simulink model "mining_feeder_layer_FDIR"  (R2024a)
settings: Solver=ode23t  StartTime=0.0  StopTime=2.0  FixedStep=5e-06  MaxStep=0.001  RelTol=1e-3
undefined symbols (not defined in the file or in its folder): D11, Delta, gcbh, Newton, Raphson, sps_rtmsupport
libraries: spsFourierLib x8, spsMeanLib x8, spsThreePhaseVIMeasurementLib x7, spsRMSLib x6, spsThreePhaseBreakerLib x5, spsThreePhaseSeriesRLCLoadLib x4, spsThreePhaseFaultLib x4, spsThreePhasePISectionLineLib x4, spsThreePhaseTransformerTwoWindingsLib x2, spsThreePhaseSourceLib x1, sps_lib x1
settings Model: Creator=victo  LastModifiedBy=victo

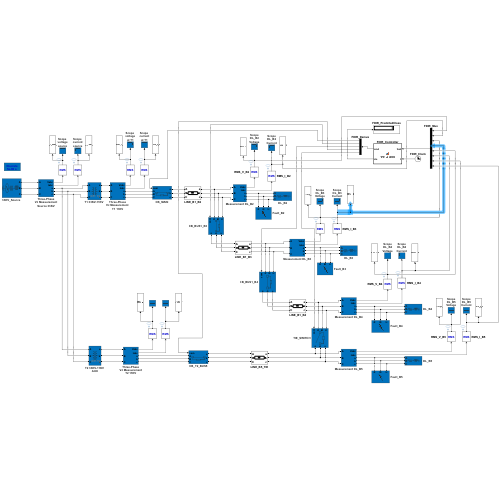
[thumbnail: Simulink's stored preview of the top-level diagram]
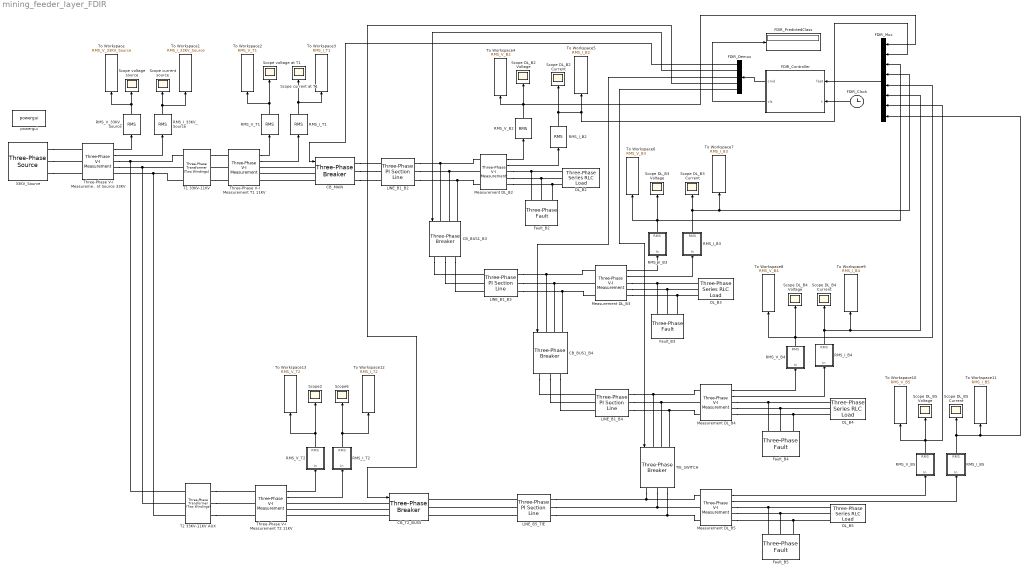
== system mining_feeder_layer_FDIR ==
  "33KV_Source " : spsThreePhaseSourceLib/Three-Phase Source  InternalConnection=Yg  VoltagePhases=off  Voltage=33e3  PhaseAngle=0  Voltage_phases=[25e3 25e3 25e3]/sqrt(3)  PhaseAngles_phases=[0 -120 +120]  Frequency=50  NonIdealSource=on  SpecifyImpedance=on  Resistance=0.8929  Inductance=16.58e-3  ShortCircuitLevel=500e6  BaseVoltage=33e3  XRratio=10  BusType=swing  Pref=10e3  Qref=0  Prefabc=[10e3, 10e3, 10e3]  Qrefabc=[0, 0, 0]  Qmin=-inf  Qmax=inf
  CB_BUS1_B3 : spsThreePhaseBreakerLib/Three-Phase Breaker  InitialState=closed  SwitchA=on  SwitchB=on  SwitchC=on  SwitchTimes=[1000000 1000001]  External=on  BreakerResistance=0.01  SnubberResistance=1e5  SnubberCapacitance=1e-9  Measurements=None
  CB_BUS1_B4 : spsThreePhaseBreakerLib/Three-Phase Breaker  InitialState=closed  SwitchA=on  SwitchB=on  SwitchC=on  SwitchTimes=[1000000 1000001]  External=on  BreakerResistance=0.01  SnubberResistance=1e5  SnubberCapacitance=1e-9  Measurements=None
  CB_MAIN : spsThreePhaseBreakerLib/Three-Phase Breaker  InitialState=closed  SwitchA=on  SwitchB=on  SwitchC=on  SwitchTimes=[1000000 1000001]  External=on  BreakerResistance=0.01  SnubberResistance=1e6  SnubberCapacitance=inf  Measurements=None
  CB_T2_BUS5 : spsThreePhaseBreakerLib/Three-Phase Breaker  InitialState=closed  SwitchA=on  SwitchB=on  SwitchC=on  SwitchTimes=[1000000 1000001]  External=on  BreakerResistance=0.01  SnubberResistance=1e5  SnubberCapacitance=1e-9  Measurements=None
  DL_B2 : spsThreePhaseSeriesRLCLoadLib/Three-Phase Series RLC Load  LConnTagsString=A|B|C  Configuration=Y (grounded)  NominalVoltage=11e3  Vabc=[1e3 1e3 1e3]  Vabcp=[1e3 1e3 1e3]  NominalFrequency=50  UnbalancedPower=off  ActivePower=2340000  InductivePower=572000  CapacitivePower=0  Pabc=[10e3 9e3 11e3]  QLabc=[100 90 110]  QCabc=[100 90 110]  Pabcp=[10e3 9e3 11e3]  QLabcp=[100 90 110]  QCabcp=[100 90 110]  Measurements=None  LoadType=constant Z
  DL_B3 : spsThreePhaseSeriesRLCLoadLib/Three-Phase Series RLC Load  LConnTagsString=A|B|C  Configuration=Y (grounded)  NominalVoltage=11e3  Vabc=[1e3 1e3 1e3]  Vabcp=[1e3 1e3 1e3]  NominalFrequency=50  UnbalancedPower=off  ActivePower=3120000  InductivePower=767000  CapacitivePower=0  Pabc=[10e3 9e3 11e3]  QLabc=[100 90 110]  QCabc=[100 90 110]  Pabcp=[10e3 9e3 11e3]  QLabcp=[100 90 110]  QCabcp=[100 90 110]  Measurements=None  LoadType=constant Z
  DL_B4 : spsThreePhaseSeriesRLCLoadLib/Three-Phase Series RLC Load  LConnTagsString=A|B|C  Configuration=Y (grounded)  NominalVoltage=11e3  Vabc=[1e3 1e3 1e3]  Vabcp=[1e3 1e3 1e3]  NominalFrequency=50  UnbalancedPower=off  ActivePower=3900000  InductivePower=962000  CapacitivePower=0  Pabc=[10e3 9e3 11e3]  QLabc=[100 90 110]  QCabc=[100 90 110]  Pabcp=[10e3 9e3 11e3]  QLabcp=[100 90 110]  QCabcp=[100 90 110]  Measurements=None  LoadType=constant Z
  DL_B5 : spsThreePhaseSeriesRLCLoadLib/Three-Phase Series RLC Load  LConnTagsString=A|B|C  Configuration=Y (grounded)  NominalVoltage=11e3  Vabc=[1e3 1e3 1e3]  Vabcp=[1e3 1e3 1e3]  NominalFrequency=50  UnbalancedPower=off  ActivePower=2574000  InductivePower=637000  CapacitivePower=0  Pabc=[10e3 9e3 11e3]  QLabc=[100 90 110]  QCabc=[100 90 110]  Pabcp=[10e3 9e3 11e3]  QLabcp=[100 90 110]  QCabcp=[100 90 110]  Measurements=None  LoadType=constant Z
  FDIR_Clock : Clock
  FDIR_Controller : MATLAB Function  TreatAsAtomicUnit=on
  FDIR_Demux : Demux  Outputs=5
  FDIR_Mux : Mux  Inputs=8
  FDIR_PredictedClass : Display
  Fault_B2 : spsThreePhaseFaultLib/Three-Phase Fault  InitialStates=0  FaultA=off  FaultB=off  FaultC=off  GroundFault=off  SwitchTimes=[100000 100001]  External=off  SwitchStatus=NaN  FaultResistance=0.001  GroundResistance=0.001  SnubberResistance=1e5  SnubberCapacitance=1e-9  Measurements=None
  Fault_B3 : spsThreePhaseFaultLib/Three-Phase Fault  InitialStates=0  FaultA=off  FaultB=off  FaultC=off  GroundFault=off  SwitchTimes=[1000000 1000001]  External=off  SwitchStatus=NaN  FaultResistance=0.001  GroundResistance=0.001  SnubberResistance=1e5  SnubberCapacitance=1e-9  Measurements=None
  Fault_B4 : spsThreePhaseFaultLib/Three-Phase Fault  InitialStates=0  FaultA=off  FaultB=off  FaultC=off  GroundFault=off  SwitchTimes=[1000000 1000001]  External=off  SwitchStatus=NaN  FaultResistance=0.001  GroundResistance=0.001  SnubberResistance=1e5  SnubberCapacitance=1e-9  Measurements=None
  Fault_B5 : spsThreePhaseFaultLib/Three-Phase Fault  InitialStates=0  FaultA=off  FaultB=off  FaultC=off  GroundFault=off  SwitchTimes=[1000000 1000001]  External=off  SwitchStatus=NaN  FaultResistance=0.001  GroundResistance=0.001  SnubberResistance=1e5  SnubberCapacitance=1e-9  Measurements=None
  LINE_B1_B2 : spsThreePhasePISectionLineLib/Three-Phase PI Section Line  LConnTagsString=a|b|c  RConnTagsString=A|B|C  Length=0.8  Frequency=50  Resistances=[0.12 0.36]  Inductances=[0.35e-3 1.05e-3]  Capacitances=[0.20e-6 0.10e-6]
  LINE_B1_B3 : spsThreePhasePISectionLineLib/Three-Phase PI Section Line  LConnTagsString=a|b|c  RConnTagsString=A|B|C  Length=1.2  Frequency=50  Resistances=[0.12 0.36]  Inductances=[0.35e-3 1.05e-3]  Capacitances=[0.20e-6 0.10e-6]
  LINE_B1_B4 : spsThreePhasePISectionLineLib/Three-Phase PI Section Line  LConnTagsString=a|b|c  RConnTagsString=A|B|C  Length=1.0  Frequency=50  Resistances=[0.12 0.36]  Inductances=[0.35e-3 1.05e-3]  Capacitances=[0.20e-6 0.10e-6]
  LINE_B5_TIE : spsThreePhasePISectionLineLib/Three-Phase PI Section Line  LConnTagsString=a|b|c  RConnTagsString=A|B|C  Length=0.6  Frequency=50  Resistances=[0.12 0.36]  Inductances=[0.35e-3 1.05e-3]  Capacitances=[0.20e-6 0.10e-6]
  Measurement DL_B{2..5} (4 alike) : spsThreePhaseVIMeasurementLib/Three-Phase V-I Measurement  VoltageMeasurement=phase-to-phase  SetLabelV=off  LabelV=Vabc  Vpu=off  VpuLL=off  CurrentMeasurement=yes  SetLabelI=off  LabelI=Iabc  Ipu=off  Pbase=100e6  Vbase=500e3  OutputType=Complex  PhasorSimulation=off  PSBequivalent=0
  RMS_I_33KV_Source : spsRMSLib/RMS  TrueRMS=on  Freq=50  RMSInit=0  Ts=0.0001
  RMS_I_B2 : spsRMSLib/RMS  TrueRMS=on  Freq=50  RMSInit=50  Ts=0.0001
  RMS_I_B3 : Subsystem  DialogController=POWERSYS.PowerSysDialog  LoadFcn=sps_rtmsupport('LoadFcn', gcbh);  StartFcn=sps_rtmsupport('StartFcn', gcbh);  StopFcn=sps_rtmsupport('StopFcn', gcbh);  mask(RMS){TrueRMS=on, Freq=50, RMSInit=0, Ts=0.0001}
      mask prompts: TrueRMS "True RMS value"; Freq "Fundamental frequency (Hz):"; RMSInit "Initial RMS value:"; Ts "Sample time:"
      mask help:
      | Measure the true root mean square (RMS) value of the input signal at the specified fundamental frequency.
      |
      | When True RMS value parameter is unchecked, the block outputs the RMS value of the fundamental component of the input signal.
      mask init:
      | [sps] = powericon('RMSInit',gcb,Freq,RMSInit,TrueRMS,Ts);
      settings: LibrarySourceBlock=sps_lib/Sensors and Measurements/RMS  CopyFcn=sps_rtmsupport('CopyFcn', gcbh);  DeleteFcn=sps_rtmsupport('DeleteFcn', gcbh);  UndoDeleteFcn=sps_rtmsupport('UndoDeleteFcn', gcbh);  ModelCloseFcn=sps_rtmsupport('ModelCloseFcn', gcbh);  PreSaveFcn=sps_rtmsupport('PreSaveFcn', gcbh);  PostSaveFcn=sps_rtmsupport('PostSaveFcn', gcbh);  NameChangeFcn=sps_rtmsupport('NameChangeFcn', gcbh);  PreCopyFcn=sps_rtmsupport('PreCopyFcn', gcbh);  OpenFcn=sps_rtmsupport('OpenFcn', gcbh, [1]);  CloseFcn=sps_rtmsupport('CloseFcn', gcbh);  PreDeleteFcn=sps_rtmsupport('PreDeleteFcn', gcbh);
      mask Help: helpview(psbhelp);
      mask Display: color('blue');disp('RMS')
  RMS_I_B4 : Subsystem  DialogController=POWERSYS.PowerSysDialog  LoadFcn=sps_rtmsupport('LoadFcn', gcbh);  StartFcn=sps_rtmsupport('StartFcn', gcbh);  StopFcn=sps_rtmsupport('StopFcn', gcbh);  mask(RMS){TrueRMS=on, Freq=50, RMSInit=0, Ts=0.0001}
      mask prompts: TrueRMS "True RMS value"; Freq "Fundamental frequency (Hz):"; RMSInit "Initial RMS value:"; Ts "Sample time:"
      mask help:
      | Measure the true root mean square (RMS) value of the input signal at the specified fundamental frequency.
      |
      | When True RMS value parameter is unchecked, the block outputs the RMS value of the fundamental component of the input signal.
      mask init:
      | [sps] = powericon('RMSInit',gcb,Freq,RMSInit,TrueRMS,Ts);
      settings: LibrarySourceBlock=sps_lib/Sensors and Measurements/RMS  CopyFcn=sps_rtmsupport('CopyFcn', gcbh);  DeleteFcn=sps_rtmsupport('DeleteFcn', gcbh);  UndoDeleteFcn=sps_rtmsupport('UndoDeleteFcn', gcbh);  ModelCloseFcn=sps_rtmsupport('ModelCloseFcn', gcbh);  PreSaveFcn=sps_rtmsupport('PreSaveFcn', gcbh);  PostSaveFcn=sps_rtmsupport('PostSaveFcn', gcbh);  NameChangeFcn=sps_rtmsupport('NameChangeFcn', gcbh);  PreCopyFcn=sps_rtmsupport('PreCopyFcn', gcbh);  OpenFcn=sps_rtmsupport('OpenFcn', gcbh, [1]);  CloseFcn=sps_rtmsupport('CloseFcn', gcbh);  PreDeleteFcn=sps_rtmsupport('PreDeleteFcn', gcbh);
      mask Help: helpview(psbhelp);
      mask Display: color('blue');disp('RMS')
  RMS_I_B5 : Subsystem  DialogController=POWERSYS.PowerSysDialog  LoadFcn=sps_rtmsupport('LoadFcn', gcbh);  StartFcn=sps_rtmsupport('StartFcn', gcbh);  StopFcn=sps_rtmsupport('StopFcn', gcbh);  mask(RMS){TrueRMS=on, Freq=50, RMSInit=0, Ts=0.0001}
      mask prompts: TrueRMS "True RMS value"; Freq "Fundamental frequency (Hz):"; RMSInit "Initial RMS value:"; Ts "Sample time:"
      mask help:
      | Measure the true root mean square (RMS) value of the input signal at the specified fundamental frequency.
      |
      | When True RMS value parameter is unchecked, the block outputs the RMS value of the fundamental component of the input signal.
      mask init:
      | [sps] = powericon('RMSInit',gcb,Freq,RMSInit,TrueRMS,Ts);
      settings: LibrarySourceBlock=sps_lib/Sensors and Measurements/RMS  CopyFcn=sps_rtmsupport('CopyFcn', gcbh);  DeleteFcn=sps_rtmsupport('DeleteFcn', gcbh);  UndoDeleteFcn=sps_rtmsupport('UndoDeleteFcn', gcbh);  ModelCloseFcn=sps_rtmsupport('ModelCloseFcn', gcbh);  PreSaveFcn=sps_rtmsupport('PreSaveFcn', gcbh);  PostSaveFcn=sps_rtmsupport('PostSaveFcn', gcbh);  NameChangeFcn=sps_rtmsupport('NameChangeFcn', gcbh);  PreCopyFcn=sps_rtmsupport('PreCopyFcn', gcbh);  OpenFcn=sps_rtmsupport('OpenFcn', gcbh, [1]);  CloseFcn=sps_rtmsupport('CloseFcn', gcbh);  PreDeleteFcn=sps_rtmsupport('PreDeleteFcn', gcbh);
      mask Help: helpview(psbhelp);
      mask Display: color('blue');disp('RMS')
  RMS_I_T1 : spsRMSLib/RMS  TrueRMS=on  Freq=50  RMSInit=0  Ts=0.0001
  RMS_I_T2 : Subsystem  DialogController=POWERSYS.PowerSysDialog  LoadFcn=sps_rtmsupport('LoadFcn', gcbh);  StartFcn=sps_rtmsupport('StartFcn', gcbh);  StopFcn=sps_rtmsupport('StopFcn', gcbh);  mask(RMS){TrueRMS=on, Freq=50, RMSInit=0, Ts=0.0001}
      mask prompts: TrueRMS "True RMS value"; Freq "Fundamental frequency (Hz):"; RMSInit "Initial RMS value:"; Ts "Sample time:"
      mask help:
      | Measure the true root mean square (RMS) value of the input signal at the specified fundamental frequency.
      |
      | When True RMS value parameter is unchecked, the block outputs the RMS value of the fundamental component of the input signal.
      mask init:
      | [sps] = powericon('RMSInit',gcb,Freq,RMSInit,TrueRMS,Ts);
      settings: LibrarySourceBlock=sps_lib/Sensors and Measurements/RMS  CopyFcn=sps_rtmsupport('CopyFcn', gcbh);  DeleteFcn=sps_rtmsupport('DeleteFcn', gcbh);  UndoDeleteFcn=sps_rtmsupport('UndoDeleteFcn', gcbh);  ModelCloseFcn=sps_rtmsupport('ModelCloseFcn', gcbh);  PreSaveFcn=sps_rtmsupport('PreSaveFcn', gcbh);  PostSaveFcn=sps_rtmsupport('PostSaveFcn', gcbh);  NameChangeFcn=sps_rtmsupport('NameChangeFcn', gcbh);  PreCopyFcn=sps_rtmsupport('PreCopyFcn', gcbh);  OpenFcn=sps_rtmsupport('OpenFcn', gcbh, [1]);  CloseFcn=sps_rtmsupport('CloseFcn', gcbh);  PreDeleteFcn=sps_rtmsupport('PreDeleteFcn', gcbh);
      mask Help: helpview(psbhelp);
      mask Display: color('blue');disp('RMS')
  RMS_V_33KV_Source : spsRMSLib/RMS  TrueRMS=on  Freq=50  RMSInit=0  Ts=0.0001
  RMS_V_B2 : spsRMSLib/RMS  TrueRMS=on  Freq=50  RMSInit=9000  Ts=0.0001
  RMS_V_B3 : Subsystem  DialogController=POWERSYS.PowerSysDialog  LoadFcn=sps_rtmsupport('LoadFcn', gcbh);  StartFcn=sps_rtmsupport('StartFcn', gcbh);  StopFcn=sps_rtmsupport('StopFcn', gcbh);  mask(RMS){TrueRMS=on, Freq=50, RMSInit=0, Ts=0.0001}
      mask prompts: TrueRMS "True RMS value"; Freq "Fundamental frequency (Hz):"; RMSInit "Initial RMS value:"; Ts "Sample time:"
      mask help:
      | Measure the true root mean square (RMS) value of the input signal at the specified fundamental frequency.
      |
      | When True RMS value parameter is unchecked, the block outputs the RMS value of the fundamental component of the input signal.
      mask init:
      | [sps] = powericon('RMSInit',gcb,Freq,RMSInit,TrueRMS,Ts);
      settings: LibrarySourceBlock=sps_lib/Sensors and Measurements/RMS  CopyFcn=sps_rtmsupport('CopyFcn', gcbh);  DeleteFcn=sps_rtmsupport('DeleteFcn', gcbh);  UndoDeleteFcn=sps_rtmsupport('UndoDeleteFcn', gcbh);  ModelCloseFcn=sps_rtmsupport('ModelCloseFcn', gcbh);  PreSaveFcn=sps_rtmsupport('PreSaveFcn', gcbh);  PostSaveFcn=sps_rtmsupport('PostSaveFcn', gcbh);  NameChangeFcn=sps_rtmsupport('NameChangeFcn', gcbh);  PreCopyFcn=sps_rtmsupport('PreCopyFcn', gcbh);  OpenFcn=sps_rtmsupport('OpenFcn', gcbh, [1]);  CloseFcn=sps_rtmsupport('CloseFcn', gcbh);  PreDeleteFcn=sps_rtmsupport('PreDeleteFcn', gcbh);
      mask Help: helpview(psbhelp);
      mask Display: color('blue');disp('RMS')
  RMS_V_B4 : Subsystem  DialogController=POWERSYS.PowerSysDialog  LoadFcn=sps_rtmsupport('LoadFcn', gcbh);  StartFcn=sps_rtmsupport('StartFcn', gcbh);  StopFcn=sps_rtmsupport('StopFcn', gcbh);  mask(RMS){TrueRMS=on, Freq=50, RMSInit=0, Ts=0.0001}
      mask prompts: TrueRMS "True RMS value"; Freq "Fundamental frequency (Hz):"; RMSInit "Initial RMS value:"; Ts "Sample time:"
      mask help:
      | Measure the true root mean square (RMS) value of the input signal at the specified fundamental frequency.
      |
      | When True RMS value parameter is unchecked, the block outputs the RMS value of the fundamental component of the input signal.
      mask init:
      | [sps] = powericon('RMSInit',gcb,Freq,RMSInit,TrueRMS,Ts);
      settings: LibrarySourceBlock=sps_lib/Sensors and Measurements/RMS  CopyFcn=sps_rtmsupport('CopyFcn', gcbh);  DeleteFcn=sps_rtmsupport('DeleteFcn', gcbh);  UndoDeleteFcn=sps_rtmsupport('UndoDeleteFcn', gcbh);  ModelCloseFcn=sps_rtmsupport('ModelCloseFcn', gcbh);  PreSaveFcn=sps_rtmsupport('PreSaveFcn', gcbh);  PostSaveFcn=sps_rtmsupport('PostSaveFcn', gcbh);  NameChangeFcn=sps_rtmsupport('NameChangeFcn', gcbh);  PreCopyFcn=sps_rtmsupport('PreCopyFcn', gcbh);  OpenFcn=sps_rtmsupport('OpenFcn', gcbh, [1]);  CloseFcn=sps_rtmsupport('CloseFcn', gcbh);  PreDeleteFcn=sps_rtmsupport('PreDeleteFcn', gcbh);
      mask Help: helpview(psbhelp);
      mask Display: color('blue');disp('RMS')
  RMS_V_B5 : Subsystem  DialogController=POWERSYS.PowerSysDialog  LoadFcn=sps_rtmsupport('LoadFcn', gcbh);  StartFcn=sps_rtmsupport('StartFcn', gcbh);  StopFcn=sps_rtmsupport('StopFcn', gcbh);  mask(RMS){TrueRMS=on, Freq=50, RMSInit=0, Ts=0.0001}
      mask prompts: TrueRMS "True RMS value"; Freq "Fundamental frequency (Hz):"; RMSInit "Initial RMS value:"; Ts "Sample time:"
      mask help:
      | Measure the true root mean square (RMS) value of the input signal at the specified fundamental frequency.
      |
      | When True RMS value parameter is unchecked, the block outputs the RMS value of the fundamental component of the input signal.
      mask init:
      | [sps] = powericon('RMSInit',gcb,Freq,RMSInit,TrueRMS,Ts);
      settings: LibrarySourceBlock=sps_lib/Sensors and Measurements/RMS  CopyFcn=sps_rtmsupport('CopyFcn', gcbh);  DeleteFcn=sps_rtmsupport('DeleteFcn', gcbh);  UndoDeleteFcn=sps_rtmsupport('UndoDeleteFcn', gcbh);  ModelCloseFcn=sps_rtmsupport('ModelCloseFcn', gcbh);  PreSaveFcn=sps_rtmsupport('PreSaveFcn', gcbh);  PostSaveFcn=sps_rtmsupport('PostSaveFcn', gcbh);  NameChangeFcn=sps_rtmsupport('NameChangeFcn', gcbh);  PreCopyFcn=sps_rtmsupport('PreCopyFcn', gcbh);  OpenFcn=sps_rtmsupport('OpenFcn', gcbh, [1]);  CloseFcn=sps_rtmsupport('CloseFcn', gcbh);  PreDeleteFcn=sps_rtmsupport('PreDeleteFcn', gcbh);
      mask Help: helpview(psbhelp);
      mask Display: color('blue');disp('RMS')
  RMS_V_T1 : spsRMSLib/RMS  TrueRMS=on  Freq=50  RMSInit=0  Ts=0.0001
  RMS_V_T2 : Subsystem  DialogController=POWERSYS.PowerSysDialog  LoadFcn=sps_rtmsupport('LoadFcn', gcbh);  StartFcn=sps_rtmsupport('StartFcn', gcbh);  StopFcn=sps_rtmsupport('StopFcn', gcbh);  mask(RMS){TrueRMS=on, Freq=50, RMSInit=0, Ts=0.0001}
      mask prompts: TrueRMS "True RMS value"; Freq "Fundamental frequency (Hz):"; RMSInit "Initial RMS value:"; Ts "Sample time:"
      mask help:
      | Measure the true root mean square (RMS) value of the input signal at the specified fundamental frequency.
      |
      | When True RMS value parameter is unchecked, the block outputs the RMS value of the fundamental component of the input signal.
      mask init:
      | [sps] = powericon('RMSInit',gcb,Freq,RMSInit,TrueRMS,Ts);
      settings: LibrarySourceBlock=sps_lib/Sensors and Measurements/RMS  CopyFcn=sps_rtmsupport('CopyFcn', gcbh);  DeleteFcn=sps_rtmsupport('DeleteFcn', gcbh);  UndoDeleteFcn=sps_rtmsupport('UndoDeleteFcn', gcbh);  ModelCloseFcn=sps_rtmsupport('ModelCloseFcn', gcbh);  PreSaveFcn=sps_rtmsupport('PreSaveFcn', gcbh);  PostSaveFcn=sps_rtmsupport('PostSaveFcn', gcbh);  NameChangeFcn=sps_rtmsupport('NameChangeFcn', gcbh);  PreCopyFcn=sps_rtmsupport('PreCopyFcn', gcbh);  OpenFcn=sps_rtmsupport('OpenFcn', gcbh, [1]);  CloseFcn=sps_rtmsupport('CloseFcn', gcbh);  PreDeleteFcn=sps_rtmsupport('PreDeleteFcn', gcbh);
      mask Help: helpview(psbhelp);
      mask Display: color('blue');disp('RMS')
  Scope DL_B2 Current : Scope
  Scope DL_B2 Voltage : Scope
  Scope DL_B3 Current : Scope
  Scope DL_B3 Voltage : Scope
  Scope DL_B4 Current : Scope
  Scope DL_B4 Voltage : Scope
  Scope DL_B5 Current : Scope
  Scope DL_B5 Voltage : Scope
  Scope current at T1 : Scope
  Scope current source : Scope
  Scope voltage at T1 : Scope
  Scope voltage source : Scope
  Scope2 : Scope
  Scope6 : Scope
  "T1 33KV-11KV " : spsThreePhaseTransformerTwoWindingsLib/Three-Phase Transformer (Two Windings)  Winding1Connection=Delta (D11)  Winding2Connection=Yg  CoreType=Three single-phase transformers  SetSaturation=off  Hysteresis=off  DataFile='hysteresis'  SetInitialFlux=off  Measurements=None  UNITS=pu  NominalPower=[ 20e6 , 50 ]  Winding1=[33e3 0.002 0.04]  Winding2=[11e3 0.002 0.04]  Rm=499.98  Lm=500  L0=0.5  Saturation=[0 0;0.0024 1.2;1 1.52]  InitialFluxes=[ 0.8 , -0.8 , 0.7 ]  BreakLoop=off  DiscreteSolver=Trapezoidal iterative  DataType=off  TransfoNumber=1
  T2 33KV-11KV AUX : spsThreePhaseTransformerTwoWindingsLib/Three-Phase Transformer (Two Windings)  Winding1Connection=Delta (D11)  Winding2Connection=Yg  CoreType=Three single-phase transformers  SetSaturation=off  Hysteresis=off  DataFile='hysteresis'  SetInitialFlux=off  Measurements=None  UNITS=pu  NominalPower=[ 15e6 , 50 ]  Winding1=[33e3 0.002 0.04]  Winding2=[11e3 0.002 0.04]  Rm=499.98  Lm=500  L0=0.5  Saturation=[0 0;0.0024 1.2;1 1.52]  InitialFluxes=[ 0.8 , -0.8 , 0.7 ]  BreakLoop=off  DiscreteSolver=Trapezoidal iterative  DataType=off  TransfoNumber=1
  TIE_SWITCH : spsThreePhaseBreakerLib/Three-Phase Breaker  InitialState=open  SwitchA=on  SwitchB=on  SwitchC=on  SwitchTimes=[1000000 1000001]  External=on  BreakerResistance=0.01  SnubberResistance=1e5  SnubberCapacitance=1e-9  Measurements=None
  Three-Phase V-I Measurement Source 33KV : spsThreePhaseVIMeasurementLib/Three-Phase V-I Measurement  VoltageMeasurement=phase-to-phase  SetLabelV=off  LabelV=Vabc  Vpu=off  VpuLL=off  CurrentMeasurement=yes  SetLabelI=off  LabelI=Iabc  Ipu=off  Pbase=100e6  Vbase=500e3  OutputType=Complex  PhasorSimulation=off  PSBequivalent=0
  Three-Phase V-I Measurement T2 11KV : spsThreePhaseVIMeasurementLib/Three-Phase V-I Measurement  VoltageMeasurement=phase-to-phase  SetLabelV=off  LabelV=Vabc  Vpu=off  VpuLL=off  CurrentMeasurement=yes  SetLabelI=off  LabelI=Iabc  Ipu=off  Pbase=100e6  Vbase=500e3  OutputType=Complex  PhasorSimulation=off  PSBequivalent=0
  Three-Phase V-I Measurement T1 11KV : spsThreePhaseVIMeasurementLib/Three-Phase V-I Measurement  VoltageMeasurement=phase-to-phase  SetLabelV=off  LabelV=Vabc  Vpu=off  VpuLL=off  CurrentMeasurement=yes  SetLabelI=off  LabelI=Iabc  Ipu=off  Pbase=100e6  Vbase=500e3  OutputType=Complex  PhasorSimulation=off  PSBequivalent=0
  To Workspace : ToWorkspace  VariableName=RMS_V_33KV_Source  SaveFormat=Structure With Time  SampleTime=-1
  To Workspace1 : ToWorkspace  VariableName=RMS_I_33KV_Source  SaveFormat=Structure With Time  SampleTime=-1
  To Workspace10 : ToWorkspace  VariableName=RMS_V_B5  SaveFormat=Structure With Time  SampleTime=-1
  To Workspace11 : ToWorkspace  VariableName=RMS_I_B5  SaveFormat=Structure With Time  SampleTime=-1
  To Workspace12 : ToWorkspace  VariableName=RMS_I_T2  SaveFormat=Structure With Time  SampleTime=-1
  To Workspace13 : ToWorkspace  VariableName=RMS_V_T2  SaveFormat=Timeseries  SampleTime=-1
  To Workspace2 : ToWorkspace  VariableName=RMS_V_T1  SaveFormat=Structure With Time  SampleTime=-1
  To Workspace3 : ToWorkspace  VariableName=RMS_I_T1  SaveFormat=Structure With Time  SampleTime=-1
  To Workspace4 : ToWorkspace  VariableName=RMS_V_B2  SaveFormat=Structure With Time  SampleTime=-1
  To Workspace5 : ToWorkspace  VariableName=RMS_I_B2  SaveFormat=Structure With Time  SampleTime=-1
  To Workspace6 : ToWorkspace  VariableName=RMS_V_B3  SaveFormat=Structure With Time  SampleTime=-1
  To Workspace7 : ToWorkspace  VariableName=RMS_I_B3  SaveFormat=Structure With Time  SampleTime=-1
  To Workspace8 : ToWorkspace  VariableName=RMS_V_B4  SaveFormat=Structure With Time  SampleTime=-1
  To Workspace9 : ToWorkspace  VariableName=RMS_I_B4  SaveFormat=Structure With Time  SampleTime=-1
  powergui : sps_lib/powergui  Priority=1  SimulationMode=Discrete  SampleTime=5e-6  frequency=60  Iterations=50  frequencyindice=50  Pbase=100e6  ErrMax=1e-4  UnitsV=kV  UnitsW=MW  buscounter=0  FunctionMessages=off  echomessages=off  EnableUseOfTLC=off  CurrentSourceSwitches=off  DisableSnubberDevices=off  DisableRonSwitches=off  DisableVfSwitches=off  DisplayEquations=off  AutomaticDiscreteSolvers=off  SolverType=Tustin/Backward Euler (TBE)  Interpol=off  ExternalGateDelay=off  methode=off  Ts=100  x0status=blocks  SPID=on  SwTol=0  HookPort=off  NonlinearTolerance=1e-4  nMaxIteration=100  ContinueOnMaxIteration=off  RestoreLinks=warning  ResistiveCurrentMeasurement=off  Frange=[0:2:500]  Ylog=off  Xlog=on  ShowGrid=off  save=off  variable=ZData  structure=0  ZoomFFT=off  StartTime=0.0  cycles=1  DisplayStyle=1  fundamental=60  FreqAxis=off  MaxFrequency=1000  frequencyindicesteady=1  RmsSteady=1  display=off
  wires:
  Measurement DL_B3/2 -> RMS_I_B3/1(In)
  Three-Phase V-I Measurement Source 33KV/2 -> RMS_I_33KV_Source/1
  Measurement DL_B4/1 -> RMS_V_B4/1(In)
  Measurement DL_B4/2 -> RMS_I_B4/1(In)
  Measurement DL_B3/1 -> RMS_V_B3/1(In)
  Three-Phase V-I Measurement T1 11KV/1 -> RMS_V_T1/1
  Three-Phase V-I Measurement T2 11KV/1 -> RMS_V_T2/1(In)
  Three-Phase V-I Measurement Source 33KV/1 -> RMS_V_33KV_Source/1
  Three-Phase V-I Measurement T2 11KV/2 -> RMS_I_T2/1(In)
  Three-Phase V-I Measurement T1 11KV/2 -> RMS_I_T1/1
  Measurement DL_B5/2 -> RMS_I_B5/1(In)
  Measurement DL_B5/1 -> RMS_V_B5/1(In)
  RMS_V_33KV_Source/1 -> Scope voltage source/1, To Workspace/1
  RMS_I_33KV_Source/1 -> Scope current source/1, To Workspace1/1
  RMS_V_B2/1 -> Scope DL_B2 Voltage/1, FDIR_Mux/1, To Workspace4/1
  RMS_V_B3/1(RMS) -> FDIR_Mux/3, To Workspace6/1, Scope DL_B3 Voltage/1
  RMS_I_B3/1(RMS) -> To Workspace7/1, FDIR_Mux/4, Scope DL_B3 Current/1
  RMS_V_B4/1(RMS) -> Scope DL_B4 Voltage/1, To Workspace8/1, FDIR_Mux/5
  RMS_I_B4/1(RMS) -> FDIR_Mux/6, To Workspace9/1, Scope DL_B4 Current/1
  RMS_V_B5/1(RMS) -> Scope DL_B5 Voltage/1, FDIR_Mux/7, To Workspace10/1
  RMS_I_B5/1(RMS) -> FDIR_Mux/8, To Workspace11/1, Scope DL_B5 Current/1
  RMS_I_B2/1 -> Scope DL_B2 Current/1, To Workspace5/1, FDIR_Mux/2
  RMS_V_T2/1(RMS) -> To Workspace13/1, Scope2/1
  RMS_V_T1/1 -> To Workspace2/1, Scope voltage at T1/1
  RMS_I_T1/1 -> To Workspace3/1, Scope current at T1/1
  Measurement DL_B2/1 -> RMS_V_B2/1
  Measurement DL_B2/2 -> RMS_I_B2/1
  RMS_I_T2/1(RMS) -> To Workspace12/1, Scope6/1
  FDIR_Mux/1 -> FDIR_Controller/1(feat)
  FDIR_Clock/1 -> FDIR_Controller/2(t)
  FDIR_Controller/2(cls) -> FDIR_PredictedClass/1
  FDIR_Demux/1 -> CB_MAIN/1
  FDIR_Demux/2 -> CB_BUS1_B3/1
  FDIR_Demux/3 -> CB_BUS1_B4/1
  FDIR_Demux/4 -> CB_T2_BUS5/1
  FDIR_Demux/5 -> TIE_SWITCH/1
  FDIR_Controller/1(cmd) -> FDIR_Demux/1
  connections:
  Three-Phase V-I Measurement Source 33KV/RConn1 -- T2 33KV-11KV AUX/LConn1 -- "T1 33KV-11KV "/LConn1
  Three-Phase V-I Measurement Source 33KV/RConn2 -- "T1 33KV-11KV "/LConn2 -- T2 33KV-11KV AUX/LConn2
  LINE_B1_B3/RConn2 -- Measurement DL_B3/LConn2 -- CB_BUS1_B4/LConn2
  LINE_B1_B3/RConn1 -- CB_BUS1_B4/LConn1 -- Measurement DL_B3/LConn1
  "33KV_Source "/RConn2 -- Three-Phase V-I Measurement Source 33KV/LConn2
  CB_BUS1_B3/LConn1 -- LINE_B1_B2/RConn1 -- Measurement DL_B2/LConn1
  Three-Phase V-I Measurement T1 11KV/LConn2 -- "T1 33KV-11KV "/RConn2
  Three-Phase V-I Measurement T1 11KV/LConn1 -- "T1 33KV-11KV "/RConn1
  Three-Phase V-I Measurement T1 11KV/LConn3 -- "T1 33KV-11KV "/RConn3
  LINE_B1_B2/RConn2 -- Measurement DL_B2/LConn2 -- CB_BUS1_B3/LConn2
  LINE_B1_B4/RConn1 -- Measurement DL_B4/LConn1 -- TIE_SWITCH/LConn1
  CB_T2_BUS5/LConn2 -- Three-Phase V-I Measurement T2 11KV/RConn2
  LINE_B1_B3/RConn3 -- Measurement DL_B3/LConn3 -- CB_BUS1_B4/LConn3
  CB_T2_BUS5/LConn1 -- Three-Phase V-I Measurement T2 11KV/RConn1
  LINE_B1_B4/RConn2 -- Measurement DL_B4/LConn2 -- TIE_SWITCH/LConn2
  LINE_B1_B2/RConn3 -- Measurement DL_B2/LConn3 -- CB_BUS1_B3/LConn3
  "33KV_Source "/RConn3 -- Three-Phase V-I Measurement Source 33KV/LConn3
  CB_T2_BUS5/LConn3 -- Three-Phase V-I Measurement T2 11KV/RConn3
  "33KV_Source "/RConn1 -- Three-Phase V-I Measurement Source 33KV/LConn1
  LINE_B1_B4/RConn3 -- Measurement DL_B4/LConn3 -- TIE_SWITCH/LConn3
  Measurement DL_B3/RConn2 -- Fault_B3/LConn2 -- DL_B3/LConn2
  Measurement DL_B3/RConn1 -- Fault_B3/LConn1 -- DL_B3/LConn1
  Measurement DL_B4/RConn1 -- Fault_B4/LConn1 -- DL_B4/LConn1
  Measurement DL_B4/RConn3 -- Fault_B4/LConn3 -- DL_B4/LConn3
  Measurement DL_B4/RConn2 -- Fault_B4/LConn2 -- DL_B4/LConn2
  Measurement DL_B5/RConn1 -- Fault_B5/LConn1 -- DL_B5/LConn1
  Measurement DL_B5/RConn2 -- Fault_B5/LConn2 -- DL_B5/LConn2
  Measurement DL_B5/RConn3 -- Fault_B5/LConn3 -- DL_B5/LConn3
  Measurement DL_B3/RConn3 -- Fault_B3/LConn3 -- DL_B3/LConn3
  CB_MAIN/RConn2 -- LINE_B1_B2/LConn2
  CB_MAIN/RConn3 -- LINE_B1_B2/LConn3
  CB_MAIN/RConn1 -- LINE_B1_B2/LConn1
  CB_MAIN/LConn1 -- Three-Phase V-I Measurement T1 11KV/RConn1
  CB_MAIN/LConn2 -- Three-Phase V-I Measurement T1 11KV/RConn2
  CB_MAIN/LConn3 -- Three-Phase V-I Measurement T1 11KV/RConn3
  "T1 33KV-11KV "/LConn3 -- T2 33KV-11KV AUX/LConn3 -- Three-Phase V-I Measurement Source 33KV/RConn3
  Measurement DL_B2/RConn2 -- Fault_B2/LConn2 -- DL_B2/LConn2
  Measurement DL_B2/RConn3 -- Fault_B2/LConn3 -- DL_B2/LConn3
  CB_BUS1_B3/RConn1 -- LINE_B1_B3/LConn1
  CB_BUS1_B3/RConn2 -- LINE_B1_B3/LConn2
  CB_BUS1_B3/RConn3 -- LINE_B1_B3/LConn3
  CB_BUS1_B4/RConn1 -- LINE_B1_B4/LConn1
  CB_BUS1_B4/RConn2 -- LINE_B1_B4/LConn2
  CB_BUS1_B4/RConn3 -- LINE_B1_B4/LConn3
  T2 33KV-11KV AUX/RConn1 -- Three-Phase V-I Measurement T2 11KV/LConn1
  T2 33KV-11KV AUX/RConn2 -- Three-Phase V-I Measurement T2 11KV/LConn2
  T2 33KV-11KV AUX/RConn3 -- Three-Phase V-I Measurement T2 11KV/LConn3
  LINE_B5_TIE/LConn2 -- CB_T2_BUS5/RConn2
  LINE_B5_TIE/LConn3 -- CB_T2_BUS5/RConn3
  LINE_B5_TIE/LConn1 -- CB_T2_BUS5/RConn1
  LINE_B5_TIE/RConn1 -- Measurement DL_B5/LConn1 -- TIE_SWITCH/RConn1
  LINE_B5_TIE/RConn2 -- Measurement DL_B5/LConn2 -- TIE_SWITCH/RConn2
  LINE_B5_TIE/RConn3 -- Measurement DL_B5/LConn3 -- TIE_SWITCH/RConn3
  Measurement DL_B2/RConn1 -- Fault_B2/LConn1 -- DL_B2/LConn1

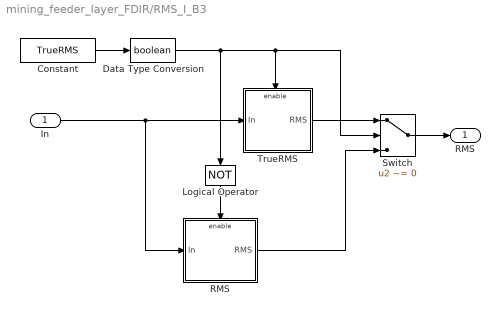
== system mining_feeder_layer_FDIR/RMS_I_B3 ==
  In : Inport  SampleTime=Ts
  Constant : Constant  Value=TrueRMS
  Data Type Conversion : DataTypeConversion  OutDataTypeStr=boolean  SaturateOnIntegerOverflow=off  RndMeth=Floor
  Logical Operator : Logic  Operator=NOT  AllPortsSameDT=off  OutDataTypeStr=boolean
  "RMS " : Subsystem
  Switch : Switch  Criteria=u2 ~= 0  Threshold=0.5  SaturateOnIntegerOverflow=off  InputSameDT=off
  "TrueRMS " : Subsystem
  RMS : Outport  SampleTime=Ts  VectorParamsAs1DForOutWhenUnconnected=off
  wires:
  Logical Operator/1 -> "RMS "/Enable
  Data Type Conversion/1 -> Switch/2, "TrueRMS "/Enable, Logical Operator/1
  Constant/1 -> Data Type Conversion/1
  "RMS "/1(RMS) -> Switch/3
  "TrueRMS "/1(RMS) -> Switch/1
  Switch/1 -> RMS/1
  In/1 -> "RMS "/1(In), "TrueRMS "/1(In)

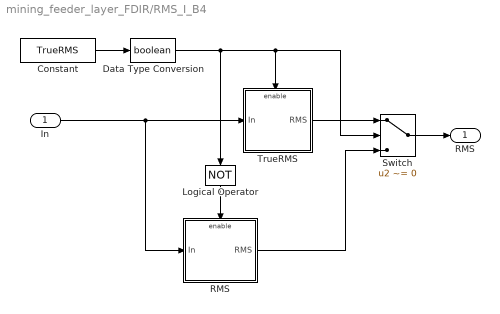
== system mining_feeder_layer_FDIR/RMS_I_B4 ==
  In : Inport  SampleTime=Ts
  Constant : Constant  Value=TrueRMS
  Data Type Conversion : DataTypeConversion  OutDataTypeStr=boolean  SaturateOnIntegerOverflow=off  RndMeth=Floor
  Logical Operator : Logic  Operator=NOT  AllPortsSameDT=off  OutDataTypeStr=boolean
  "RMS " : Subsystem
  Switch : Switch  Criteria=u2 ~= 0  Threshold=0.5  SaturateOnIntegerOverflow=off  InputSameDT=off
  "TrueRMS " : Subsystem
  RMS : Outport  SampleTime=Ts  VectorParamsAs1DForOutWhenUnconnected=off
  wires:
  Logical Operator/1 -> "RMS "/Enable
  Data Type Conversion/1 -> Switch/2, "TrueRMS "/Enable, Logical Operator/1
  Constant/1 -> Data Type Conversion/1
  "RMS "/1(RMS) -> Switch/3
  "TrueRMS "/1(RMS) -> Switch/1
  Switch/1 -> RMS/1
  In/1 -> "RMS "/1(In), "TrueRMS "/1(In)

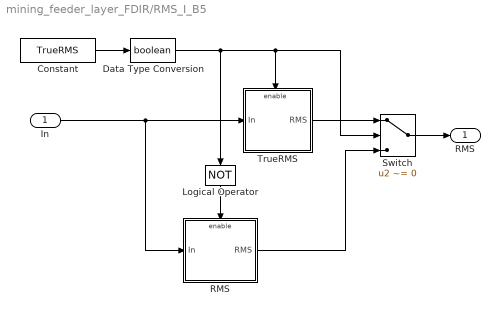
== system mining_feeder_layer_FDIR/RMS_I_B5 ==
  In : Inport  SampleTime=Ts
  Constant : Constant  Value=TrueRMS
  Data Type Conversion : DataTypeConversion  OutDataTypeStr=boolean  SaturateOnIntegerOverflow=off  RndMeth=Floor
  Logical Operator : Logic  Operator=NOT  AllPortsSameDT=off  OutDataTypeStr=boolean
  "RMS " : Subsystem
  Switch : Switch  Criteria=u2 ~= 0  Threshold=0.5  SaturateOnIntegerOverflow=off  InputSameDT=off
  "TrueRMS " : Subsystem
  RMS : Outport  SampleTime=Ts  VectorParamsAs1DForOutWhenUnconnected=off
  wires:
  Logical Operator/1 -> "RMS "/Enable
  Data Type Conversion/1 -> Switch/2, "TrueRMS "/Enable, Logical Operator/1
  Constant/1 -> Data Type Conversion/1
  "RMS "/1(RMS) -> Switch/3
  "TrueRMS "/1(RMS) -> Switch/1
  Switch/1 -> RMS/1
  In/1 -> "RMS "/1(In), "TrueRMS "/1(In)

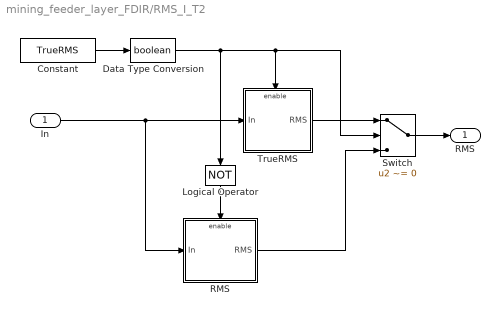
== system mining_feeder_layer_FDIR/RMS_I_T2 ==
  In : Inport  SampleTime=Ts
  Constant : Constant  Value=TrueRMS
  Data Type Conversion : DataTypeConversion  OutDataTypeStr=boolean  SaturateOnIntegerOverflow=off  RndMeth=Floor
  Logical Operator : Logic  Operator=NOT  AllPortsSameDT=off  OutDataTypeStr=boolean
  "RMS " : Subsystem
  Switch : Switch  Criteria=u2 ~= 0  Threshold=0.5  SaturateOnIntegerOverflow=off  InputSameDT=off
  "TrueRMS " : Subsystem
  RMS : Outport  SampleTime=Ts  VectorParamsAs1DForOutWhenUnconnected=off
  wires:
  Logical Operator/1 -> "RMS "/Enable
  Data Type Conversion/1 -> Switch/2, "TrueRMS "/Enable, Logical Operator/1
  Constant/1 -> Data Type Conversion/1
  "RMS "/1(RMS) -> Switch/3
  "TrueRMS "/1(RMS) -> Switch/1
  Switch/1 -> RMS/1
  In/1 -> "RMS "/1(In), "TrueRMS "/1(In)

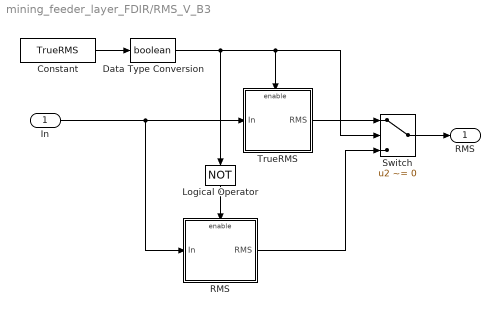
== system mining_feeder_layer_FDIR/RMS_V_B3 ==
  In : Inport  SampleTime=Ts
  Constant : Constant  Value=TrueRMS
  Data Type Conversion : DataTypeConversion  OutDataTypeStr=boolean  SaturateOnIntegerOverflow=off  RndMeth=Floor
  Logical Operator : Logic  Operator=NOT  AllPortsSameDT=off  OutDataTypeStr=boolean
  "RMS " : Subsystem
  Switch : Switch  Criteria=u2 ~= 0  Threshold=0.5  SaturateOnIntegerOverflow=off  InputSameDT=off
  "TrueRMS " : Subsystem
  RMS : Outport  SampleTime=Ts  VectorParamsAs1DForOutWhenUnconnected=off
  wires:
  Logical Operator/1 -> "RMS "/Enable
  Data Type Conversion/1 -> Switch/2, "TrueRMS "/Enable, Logical Operator/1
  Constant/1 -> Data Type Conversion/1
  "RMS "/1(RMS) -> Switch/3
  "TrueRMS "/1(RMS) -> Switch/1
  Switch/1 -> RMS/1
  In/1 -> "RMS "/1(In), "TrueRMS "/1(In)

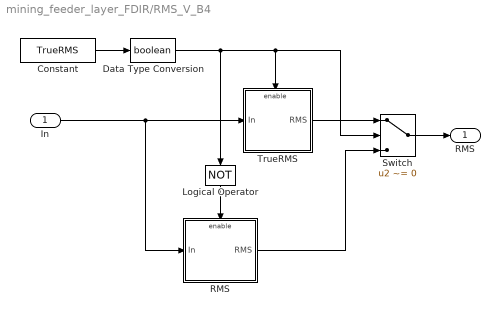
== system mining_feeder_layer_FDIR/RMS_V_B4 ==
  In : Inport  SampleTime=Ts
  Constant : Constant  Value=TrueRMS
  Data Type Conversion : DataTypeConversion  OutDataTypeStr=boolean  SaturateOnIntegerOverflow=off  RndMeth=Floor
  Logical Operator : Logic  Operator=NOT  AllPortsSameDT=off  OutDataTypeStr=boolean
  "RMS " : Subsystem
  Switch : Switch  Criteria=u2 ~= 0  Threshold=0.5  SaturateOnIntegerOverflow=off  InputSameDT=off
  "TrueRMS " : Subsystem
  RMS : Outport  SampleTime=Ts  VectorParamsAs1DForOutWhenUnconnected=off
  wires:
  Logical Operator/1 -> "RMS "/Enable
  Data Type Conversion/1 -> Switch/2, "TrueRMS "/Enable, Logical Operator/1
  Constant/1 -> Data Type Conversion/1
  "RMS "/1(RMS) -> Switch/3
  "TrueRMS "/1(RMS) -> Switch/1
  Switch/1 -> RMS/1
  In/1 -> "RMS "/1(In), "TrueRMS "/1(In)

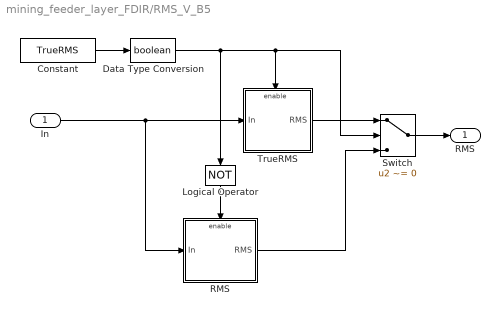
== system mining_feeder_layer_FDIR/RMS_V_B5 ==
  In : Inport  SampleTime=Ts
  Constant : Constant  Value=TrueRMS
  Data Type Conversion : DataTypeConversion  OutDataTypeStr=boolean  SaturateOnIntegerOverflow=off  RndMeth=Floor
  Logical Operator : Logic  Operator=NOT  AllPortsSameDT=off  OutDataTypeStr=boolean
  "RMS " : Subsystem
  Switch : Switch  Criteria=u2 ~= 0  Threshold=0.5  SaturateOnIntegerOverflow=off  InputSameDT=off
  "TrueRMS " : Subsystem
  RMS : Outport  SampleTime=Ts  VectorParamsAs1DForOutWhenUnconnected=off
  wires:
  Logical Operator/1 -> "RMS "/Enable
  Data Type Conversion/1 -> Switch/2, "TrueRMS "/Enable, Logical Operator/1
  Constant/1 -> Data Type Conversion/1
  "RMS "/1(RMS) -> Switch/3
  "TrueRMS "/1(RMS) -> Switch/1
  Switch/1 -> RMS/1
  In/1 -> "RMS "/1(In), "TrueRMS "/1(In)

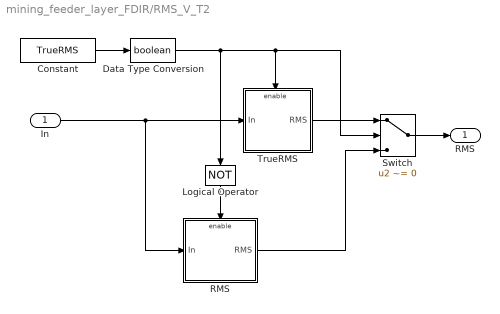
== system mining_feeder_layer_FDIR/RMS_V_T2 ==
  In : Inport  SampleTime=Ts
  Constant : Constant  Value=TrueRMS
  Data Type Conversion : DataTypeConversion  OutDataTypeStr=boolean  SaturateOnIntegerOverflow=off  RndMeth=Floor
  Logical Operator : Logic  Operator=NOT  AllPortsSameDT=off  OutDataTypeStr=boolean
  "RMS " : Subsystem
  Switch : Switch  Criteria=u2 ~= 0  Threshold=0.5  SaturateOnIntegerOverflow=off  InputSameDT=off
  "TrueRMS " : Subsystem
  RMS : Outport  SampleTime=Ts  VectorParamsAs1DForOutWhenUnconnected=off
  wires:
  Logical Operator/1 -> "RMS "/Enable
  Data Type Conversion/1 -> Switch/2, "TrueRMS "/Enable, Logical Operator/1
  Constant/1 -> Data Type Conversion/1
  "RMS "/1(RMS) -> Switch/3
  "TrueRMS "/1(RMS) -> Switch/1
  Switch/1 -> RMS/1
  In/1 -> "RMS "/1(In), "TrueRMS "/1(In)

== system mining_feeder_layer_FDIR/RMS_I_B3/RMS  ==
  In : Inport
  Enable : EnablePort
  Fourier1 : spsFourierLib/Fourier  Freq=sps.Freq  n=1  InInit=sps.Par_Init_RMS  Ts=Ts
  Gain : Gain  Gain=1/sqrt(2)
  Terminator : Terminator
  RMS : Outport  VectorParamsAs1DForOutWhenUnconnected=off
  wires:
  Gain/1 -> RMS/1
  In/1 -> Fourier1/1
  Fourier1/2 -> Terminator/1
  Fourier1/1 -> Gain/1

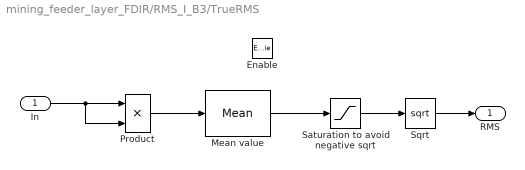
== system mining_feeder_layer_FDIR/RMS_I_B3/TrueRMS  ==
  In : Inport
  Enable : EnablePort
  Mean value : spsMeanLib/Mean  Freq=sps.Freq  Vinit=sps.Par_Init_TrueRMS  Ts=Ts
  Product : Product  InputSameDT=on  SaturateOnIntegerOverflow=on  OutDataTypeStr=Inherit: Same as first input
  Saturation to avoid negative sqrt : Saturate  UpperLimit=Inf  LowerLimit=0
  Sqrt : Sqrt  AlgorithmType=Newton-Raphson
  RMS : Outport  VectorParamsAs1DForOutWhenUnconnected=off
  wires:
  Sqrt/1 -> RMS/1
  In/1 -> Product/1, Product/2
  Product/1 -> Mean value/1
  Mean value/1 -> Saturation to avoid negative sqrt/1
  Saturation to avoid negative sqrt/1 -> Sqrt/1

== system mining_feeder_layer_FDIR/RMS_I_B4/RMS  ==
  In : Inport
  Enable : EnablePort
  Fourier1 : spsFourierLib/Fourier  Freq=sps.Freq  n=1  InInit=sps.Par_Init_RMS  Ts=Ts
  Gain : Gain  Gain=1/sqrt(2)
  Terminator : Terminator
  RMS : Outport  VectorParamsAs1DForOutWhenUnconnected=off
  wires:
  Gain/1 -> RMS/1
  In/1 -> Fourier1/1
  Fourier1/2 -> Terminator/1
  Fourier1/1 -> Gain/1

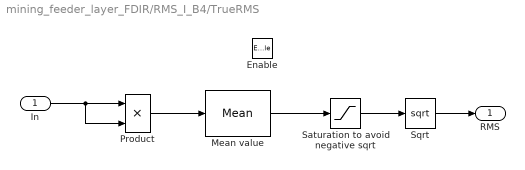
== system mining_feeder_layer_FDIR/RMS_I_B4/TrueRMS  ==
  In : Inport
  Enable : EnablePort
  Mean value : spsMeanLib/Mean  Freq=sps.Freq  Vinit=sps.Par_Init_TrueRMS  Ts=Ts
  Product : Product  InputSameDT=on  SaturateOnIntegerOverflow=on  OutDataTypeStr=Inherit: Same as first input
  Saturation to avoid negative sqrt : Saturate  UpperLimit=Inf  LowerLimit=0
  Sqrt : Sqrt  AlgorithmType=Newton-Raphson
  RMS : Outport  VectorParamsAs1DForOutWhenUnconnected=off
  wires:
  Sqrt/1 -> RMS/1
  In/1 -> Product/1, Product/2
  Product/1 -> Mean value/1
  Mean value/1 -> Saturation to avoid negative sqrt/1
  Saturation to avoid negative sqrt/1 -> Sqrt/1

== system mining_feeder_layer_FDIR/RMS_I_B5/RMS  ==
  In : Inport
  Enable : EnablePort
  Fourier1 : spsFourierLib/Fourier  Freq=sps.Freq  n=1  InInit=sps.Par_Init_RMS  Ts=Ts
  Gain : Gain  Gain=1/sqrt(2)
  Terminator : Terminator
  RMS : Outport  VectorParamsAs1DForOutWhenUnconnected=off
  wires:
  Gain/1 -> RMS/1
  In/1 -> Fourier1/1
  Fourier1/2 -> Terminator/1
  Fourier1/1 -> Gain/1

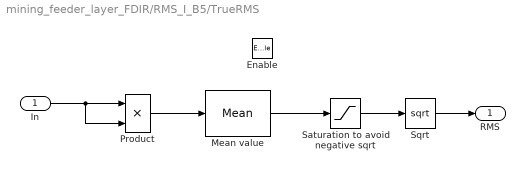
== system mining_feeder_layer_FDIR/RMS_I_B5/TrueRMS  ==
  In : Inport
  Enable : EnablePort
  Mean value : spsMeanLib/Mean  Freq=sps.Freq  Vinit=sps.Par_Init_TrueRMS  Ts=Ts
  Product : Product  InputSameDT=on  SaturateOnIntegerOverflow=on  OutDataTypeStr=Inherit: Same as first input
  Saturation to avoid negative sqrt : Saturate  UpperLimit=Inf  LowerLimit=0
  Sqrt : Sqrt  AlgorithmType=Newton-Raphson
  RMS : Outport  VectorParamsAs1DForOutWhenUnconnected=off
  wires:
  Sqrt/1 -> RMS/1
  In/1 -> Product/1, Product/2
  Product/1 -> Mean value/1
  Mean value/1 -> Saturation to avoid negative sqrt/1
  Saturation to avoid negative sqrt/1 -> Sqrt/1

== system mining_feeder_layer_FDIR/RMS_I_T2/RMS  ==
  In : Inport
  Enable : EnablePort
  Fourier1 : spsFourierLib/Fourier  Freq=sps.Freq  n=1  InInit=sps.Par_Init_RMS  Ts=Ts
  Gain : Gain  Gain=1/sqrt(2)
  Terminator : Terminator
  RMS : Outport  VectorParamsAs1DForOutWhenUnconnected=off
  wires:
  Gain/1 -> RMS/1
  In/1 -> Fourier1/1
  Fourier1/2 -> Terminator/1
  Fourier1/1 -> Gain/1

== system mining_feeder_layer_FDIR/RMS_I_T2/TrueRMS  ==
  In : Inport
  Enable : EnablePort
  Mean value : spsMeanLib/Mean  Freq=sps.Freq  Vinit=sps.Par_Init_TrueRMS  Ts=Ts
  Product : Product  InputSameDT=on  SaturateOnIntegerOverflow=on  OutDataTypeStr=Inherit: Same as first input
  Saturation to avoid negative sqrt : Saturate  UpperLimit=Inf  LowerLimit=0
  Sqrt : Sqrt  AlgorithmType=Newton-Raphson
  RMS : Outport  VectorParamsAs1DForOutWhenUnconnected=off
  wires:
  Sqrt/1 -> RMS/1
  In/1 -> Product/1, Product/2
  Product/1 -> Mean value/1
  Mean value/1 -> Saturation to avoid negative sqrt/1
  Saturation to avoid negative sqrt/1 -> Sqrt/1

== system mining_feeder_layer_FDIR/RMS_V_B3/RMS  ==
  In : Inport
  Enable : EnablePort
  Fourier1 : spsFourierLib/Fourier  Freq=sps.Freq  n=1  InInit=sps.Par_Init_RMS  Ts=Ts
  Gain : Gain  Gain=1/sqrt(2)
  Terminator : Terminator
  RMS : Outport  VectorParamsAs1DForOutWhenUnconnected=off
  wires:
  Gain/1 -> RMS/1
  In/1 -> Fourier1/1
  Fourier1/2 -> Terminator/1
  Fourier1/1 -> Gain/1

== system mining_feeder_layer_FDIR/RMS_V_B3/TrueRMS  ==
  In : Inport
  Enable : EnablePort
  Mean value : spsMeanLib/Mean  Freq=sps.Freq  Vinit=sps.Par_Init_TrueRMS  Ts=Ts
  Product : Product  InputSameDT=on  SaturateOnIntegerOverflow=on  OutDataTypeStr=Inherit: Same as first input
  Saturation to avoid negative sqrt : Saturate  UpperLimit=Inf  LowerLimit=0
  Sqrt : Sqrt  AlgorithmType=Newton-Raphson
  RMS : Outport  VectorParamsAs1DForOutWhenUnconnected=off
  wires:
  Sqrt/1 -> RMS/1
  In/1 -> Product/1, Product/2
  Product/1 -> Mean value/1
  Mean value/1 -> Saturation to avoid negative sqrt/1
  Saturation to avoid negative sqrt/1 -> Sqrt/1

== system mining_feeder_layer_FDIR/RMS_V_B4/RMS  ==
  In : Inport
  Enable : EnablePort
  Fourier1 : spsFourierLib/Fourier  Freq=sps.Freq  n=1  InInit=sps.Par_Init_RMS  Ts=Ts
  Gain : Gain  Gain=1/sqrt(2)
  Terminator : Terminator
  RMS : Outport  VectorParamsAs1DForOutWhenUnconnected=off
  wires:
  Gain/1 -> RMS/1
  In/1 -> Fourier1/1
  Fourier1/2 -> Terminator/1
  Fourier1/1 -> Gain/1

== system mining_feeder_layer_FDIR/RMS_V_B4/TrueRMS  ==
  In : Inport
  Enable : EnablePort
  Mean value : spsMeanLib/Mean  Freq=sps.Freq  Vinit=sps.Par_Init_TrueRMS  Ts=Ts
  Product : Product  InputSameDT=on  SaturateOnIntegerOverflow=on  OutDataTypeStr=Inherit: Same as first input
  Saturation to avoid negative sqrt : Saturate  UpperLimit=Inf  LowerLimit=0
  Sqrt : Sqrt  AlgorithmType=Newton-Raphson
  RMS : Outport  VectorParamsAs1DForOutWhenUnconnected=off
  wires:
  Sqrt/1 -> RMS/1
  In/1 -> Product/1, Product/2
  Product/1 -> Mean value/1
  Mean value/1 -> Saturation to avoid negative sqrt/1
  Saturation to avoid negative sqrt/1 -> Sqrt/1

== system mining_feeder_layer_FDIR/RMS_V_B5/RMS  ==
  In : Inport
  Enable : EnablePort
  Fourier1 : spsFourierLib/Fourier  Freq=sps.Freq  n=1  InInit=sps.Par_Init_RMS  Ts=Ts
  Gain : Gain  Gain=1/sqrt(2)
  Terminator : Terminator
  RMS : Outport  VectorParamsAs1DForOutWhenUnconnected=off
  wires:
  Gain/1 -> RMS/1
  In/1 -> Fourier1/1
  Fourier1/2 -> Terminator/1
  Fourier1/1 -> Gain/1

== system mining_feeder_layer_FDIR/RMS_V_B5/TrueRMS  ==
  In : Inport
  Enable : EnablePort
  Mean value : spsMeanLib/Mean  Freq=sps.Freq  Vinit=sps.Par_Init_TrueRMS  Ts=Ts
  Product : Product  InputSameDT=on  SaturateOnIntegerOverflow=on  OutDataTypeStr=Inherit: Same as first input
  Saturation to avoid negative sqrt : Saturate  UpperLimit=Inf  LowerLimit=0
  Sqrt : Sqrt  AlgorithmType=Newton-Raphson
  RMS : Outport  VectorParamsAs1DForOutWhenUnconnected=off
  wires:
  Sqrt/1 -> RMS/1
  In/1 -> Product/1, Product/2
  Product/1 -> Mean value/1
  Mean value/1 -> Saturation to avoid negative sqrt/1
  Saturation to avoid negative sqrt/1 -> Sqrt/1

== system mining_feeder_layer_FDIR/RMS_V_T2/RMS  ==
  In : Inport
  Enable : EnablePort
  Fourier1 : spsFourierLib/Fourier  Freq=sps.Freq  n=1  InInit=sps.Par_Init_RMS  Ts=Ts
  Gain : Gain  Gain=1/sqrt(2)
  Terminator : Terminator
  RMS : Outport  VectorParamsAs1DForOutWhenUnconnected=off
  wires:
  Gain/1 -> RMS/1
  In/1 -> Fourier1/1
  Fourier1/2 -> Terminator/1
  Fourier1/1 -> Gain/1

== system mining_feeder_layer_FDIR/RMS_V_T2/TrueRMS  ==
  In : Inport
  Enable : EnablePort
  Mean value : spsMeanLib/Mean  Freq=sps.Freq  Vinit=sps.Par_Init_TrueRMS  Ts=Ts
  Product : Product  InputSameDT=on  SaturateOnIntegerOverflow=on  OutDataTypeStr=Inherit: Same as first input
  Saturation to avoid negative sqrt : Saturate  UpperLimit=Inf  LowerLimit=0
  Sqrt : Sqrt  AlgorithmType=Newton-Raphson
  RMS : Outport  VectorParamsAs1DForOutWhenUnconnected=off
  wires:
  Sqrt/1 -> RMS/1
  In/1 -> Product/1, Product/2
  Product/1 -> Mean value/1
  Mean value/1 -> Saturation to avoid negative sqrt/1
  Saturation to avoid negative sqrt/1 -> Sqrt/1

== matlab function mining_feeder_layer_FDIR/FDIR_Controller ==
  data: feat input; cmd output; t input; cls output
function [cmd, cls] = FDIR_Controller(feat, t) %#codegen
% Autonomous FDIR: detect a disturbance, wait 0.5 s, classify with the trained
% Random Forest, then latch the breaker/tie commands.
%   feat: 24 RMS features [V_B2abc I_B2abc V_B3abc I_B3abc V_B4abc I_B4abc V_B5abc I_B5abc]
%   cmd : [CB_MAIN CB_BUS1_B3 CB_BUS1_B4 CB_T2_BUS5 TIE]  (1=closed, 0=open; TIE 1=closed)
coder.extrinsic('classifyRF','reportFDIR');
persistent baseI det tdet decided cmdL clsL
if isempty(det)
    baseI = ones(1,12); det = false; tdet = 0; decided = false;
    cmdL = [1 1 1 1 0]; clsL = 0;   % normal: CB closed, tie open; idle = Healthy(0)
end
f = feat(:).';
Iidx = [4 5 6 10 11 12 16 17 18 22 23 24];
Vidx = [1 2 3 7 8 9 13 14 15 19 20 21];
VBASE = 11000;
if t < 0.45
    baseI = f(Iidx);           % track the healthy pre-fault current baseline
end
if ~det && t > 0.45
    if any(f(Iidx) > 1.5*max(baseI,1)) || any(f(Vidx) < 0.85*VBASE)
        det = true; tdet = t;  % disturbance detected
    end
end
if det && ~decided && t >= tdet + 0.5
    c = 0;
    c = classifyRF(f);   % RF: 0 Healthy | 1-3 B2 | 4-6 B3 | 7-9 B4 | 10-12 B5
    clsL = c; cmdL = policy(c); decided = true;
    reportFDIR(t, c);    % prints the readable label in the Command Window
end
cmd = cmdL;
cls = clsL;
end

function cmd = policy(cls)
cmd = [1 1 1 1 0];
if cls>=1 && cls<=3        % B2: isolate (open CB_MAIN+CB_BUS1_B3), restore via tie
    cmd = [0 0 1 1 1];
elseif cls>=4 && cls<=6    % B3: isolate (open CB_BUS1_B3+CB_BUS1_B4), restore via tie
    cmd = [1 0 0 1 1];
elseif cls>=7 && cls<=9    % B4: isolate (open CB_BUS1_B4), tie stays open
    cmd = [1 1 0 1 0];
elseif cls>=10 && cls<=12  % B5: isolate (open CB_T2_BUS5), tie stays open
    cmd = [1 1 1 0 0];
end
end
